simulink model "Modelo_sensores_reales_con_Kalman_discreto"  (R2021a)
settings: Solver=ode15s  StartTime=0.0  StopTime=7  FixedStep=0.0001  RelTol=1e-5
values from neighbouring files (symbols this model uses):
  A_d1 = (eye(4)+0.5*A*T_s)*(eye(4)-0.5*A*T_s)^(-1)    [Parametros.m]
  alpha = 0.5    [Parametros.m]
  Bu_d1 = B_d1(:,1)    [Parametros.m]
  C_d1 = C1    [Parametros.m]
  Cc = 1000    [Parametros.m]
  Cmax = 900    [Parametros.m]
  Cmin = 100    [Parametros.m]
  Du_d1 = D_d1(:,1)    [Parametros.m]
  Kc = 16000    [Parametros.m]
  Kr = 160000    [Parametros.m]
  Mc = 250    [Parametros.m]
  Mr = 45    [Parametros.m]
  R_d1 = R/T_s    [Parametros.m]
  T_s = 0.0001    [Parametros.m]
undefined symbols (not defined in the file or in its folder): Discrete, sigbuilder_block, Time
libraries: ctrlSharedLib x1
settings Model: Creator=fhlla  LastModifiedBy=fhlla
settings SolverCC: ZeroCrossAlgorithm=Adaptive
settings DebuggingCC: IgnoredZcDiagnostic=none

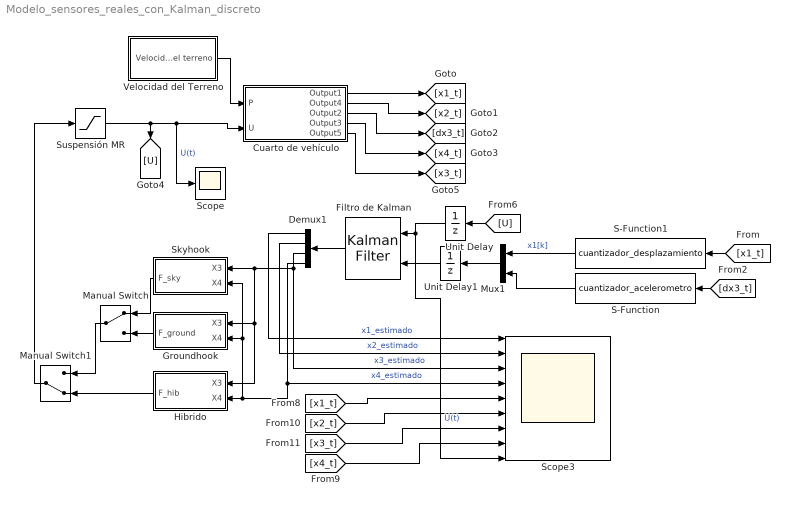
== system Modelo_sensores_reales_con_Kalman_discreto ==
  Cuarto de vehículo : Subsystem
  Demux1 : Demux
  Filtro de Kalman : ctrlSharedLib/Kalman Filter  TimeDomain=Discrete-Time  UseCurrentEstimator=on  ModelSource=Individual A, B, C, D matrices  ModelSourceVariable=ss(0.95,1,1,0,1)  A=A_d1  B=Bu_d1  C=C_d1  D=Du_d1  NumberOfStates=1  NumberOfInputs=1  NumberOfOutputs=1  InitialEstimateSource=Dialog  X0=0  P0=10  UseK=off  UseGH=off  NumberOfProcessNoiseInputs=1  G=1  TimeInvariantG=on  H=0  TimeInvariantH=on  Q=Q_d1  TimeInvariantQ=on  R=R_d1  TimeInvariantR=on  N=0  TimeInvariantN=on  AddInputPort=on  AddEnablePort=off  OutputEstimatedY=off  OutputP=off  Ts=T_s
  Groundhook : Subsystem
  Hibrido : Subsystem
  Manual Switch : ManualSwitch
  Manual Switch1 : ManualSwitch  CurrentSetting=0
  Mux1 : Mux  Inputs=2
  S-Function : S-Function  FunctionName=cuantizador_acelerometro  SFunctionDeploymentMode=off  EnableBusSupport=off
  S-Function1 : S-Function  FunctionName=cuantizador_desplazamiento  SFunctionDeploymentMode=off  EnableBusSupport=off
  Scope : Scope
  Scope3 : Scope  NumInputPorts=9
  Skyhook : Subsystem
  Suspensión MR : Saturate  UpperLimit=1500  LowerLimit=-1800
  Unit Delay : UnitDelay  SampleTime=T_s  HasFrameUpgradeWarning=on
  Unit Delay1 : UnitDelay  SampleTime=T_s  HasFrameUpgradeWarning=on
  Velocidad del Terreno : Subsystem  Tag=STV Subsys  LoadFcn=sigbuilder_block('load');  StartFcn=sigbuilder_block('start');  StopFcn=sigbuilder_block('stop');  ClipboardFcn=sigbuilder_block('clipboard');  mask(Sigbuilder block){tuvar=[0:10]}
      mask help: Simulink:masks:SigbuilderBlock_MD
      mask init:
      | if ~strcmp(get_param(bdroot(gcbh),'SimulationStatus'),'stopped') tuvar = sigbuilder_block('maskInit'); end
      settings: CopyFcn=sigbuilder_block('copy');  DeleteFcn=sigbuilder_block('delete');  ModelCloseFcn=sigbuilder_block('modelClose');  PreSaveFcn=sigbuilder_block('preSave');  PauseFcn=sigbuilder_block('pause');  ContinueFcn=sigbuilder_block('continue');  NameChangeFcn=sigbuilder_block('namechange');  OpenFcn=sigbuilder_block('open',[0 30 1024.5 488.25 ]);  CloseFcn=sigbuilder_block('close');
      mask Display: plot(0, 0, 100, 100,[2, 2, 32, 32, 2], [68, 8, 8, 68, 68],[32, 2], [38, 38], [32, 19, 2],[53, 60, 44], [32, 17, 17, 2],[16, 16, 31, 31]);txt = getActiveGroup(gcbh);text(2, 100, txt,'verticalAlignment', 'top');
  wires:
  Skyhook/1(F_sky) -> Manual Switch/1
  Groundhook/1(F_ground) -> Manual Switch/2
  Manual Switch/1 -> Manual Switch1/1
  Cuarto de vehículo/1(Output1) -> [x1_t]
  Cuarto de vehículo/2(Output4) -> [x2_t]
  Cuarto de vehículo/3(Output2) -> [dx3_t]
  S-Function1/1 -> Mux1/1  "x1[k]"
  [x1_t] -> S-Function1/1
  Cuarto de vehículo/5(Output5) -> [x3_t]
  Cuarto de vehículo/4(Output3) -> [x4_t]
  Velocidad del Terreno/1(Velocidad del terreno) -> Cuarto de vehículo/1(P)
  Hibrido/1(F_hib) -> Manual Switch1/2
  Manual Switch1/1 -> Suspensión MR/1
  [dx3_t] -> S-Function/1
  S-Function/1 -> Mux1/2
  Demux1/1 -> Scope3/1  "x1_estimado"
  Demux1/2 -> Scope3/2  "x2_estimado"
  Demux1/3 -> Scope3/3, Skyhook/1(X3), Hibrido/1(X3), Groundhook/1(X3)  "x3_estimado"
  Demux1/4 -> Hibrido/2(X4), Skyhook/2(X4), Groundhook/2(X4), Scope3/4  "x4_estimado"
  Mux1/1 -> Unit Delay1/1
  [x1_t] -> Scope3/5
  [x2_t] -> Scope3/6
  [x3_t] -> Scope3/7
  [x4_t] -> Scope3/8
  Filtro de Kalman/1 -> Demux1/1
  Unit Delay/1 -> Filtro de Kalman/1, Scope3/9  "U(t)"
  Unit Delay1/1 -> Filtro de Kalman/2
  [U] -> Unit Delay/1
  Suspensión MR/1 -> Cuarto de vehículo/2(U), Scope/1, [U]  "U(t)"

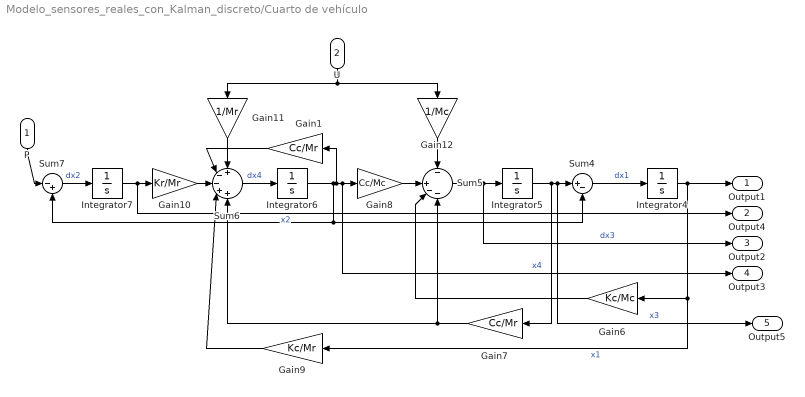
== system Modelo_sensores_reales_con_Kalman_discreto/Cuarto de vehículo ==
  P : Inport
  U : Inport  Port=2
  Gain1 : Gain  Gain=Cc/Mr
  Gain10 : Gain  Gain=Kr/Mr
  Gain11 : Gain  Gain=1/Mr
  Gain12 : Gain  Gain=1/Mc
  Gain6 : Gain  Gain=Kc/Mc
  Gain7 : Gain  Gain=Cc/Mr
  Gain8 : Gain  Gain=Cc/Mc
  Gain9 : Gain  Gain=Kc/Mr
  Integrator{4..7} (4 alike) : Integrator
  Sum4 : Sum  Inputs=|+-
  Sum5 : Sum  Inputs=-|+--
  Sum6 : Sum  Inputs=+--++
  Sum7 : Sum  Inputs=|-+
  Output1 : Outport
  Output4 : Outport  Port=2
  Output2 : Outport  Port=3
  Output3 : Outport  Port=4
  Output5 : Outport  Port=5
  wires:
  Sum7/1 -> Integrator7/1  "dx2"
  Sum6/1 -> Integrator6/1  "dx4"
  Gain9/1 -> Sum6/4
  Sum4/1 -> Integrator4/1  "dx1"
  U/1 -> Gain12/1, Gain11/1
  Sum5/1 -> Output2/1, Integrator5/1  "dx3"
  Integrator4/1 -> Gain9/1, Gain6/1, Output1/1  "x1"
  Gain10/1 -> Sum6/3
  Gain7/1 -> Sum6/5, Sum5/4
  P/1 -> Sum7/1
  Gain12/1 -> Sum5/1
  Integrator6/1 -> Gain1/1, Output3/1, Gain8/1, Sum7/2, Sum4/2  "x4"
  Integrator7/1 -> Output4/1, Gain10/1  "x2"
  Gain8/1 -> Sum5/2
  Integrator5/1 -> Output5/1, Sum4/1, Gain7/1  "x3"
  Gain1/1 -> Sum6/2
  Gain6/1 -> Sum5/3
  Gain11/1 -> Sum6/1

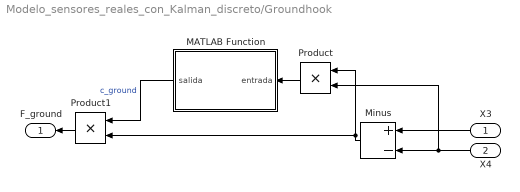
== system Modelo_sensores_reales_con_Kalman_discreto/Groundhook ==
  X3 : Inport
  X4 : Inport  Port=2
  MATLAB Function : MATLAB Function  TreatAsAtomicUnit=on
  Minus : Sum  Inputs=+-
  Product : Product
  Product1 : Product
  F_ground : Outport
  wires:
  Product/1 -> MATLAB Function/1(entrada)
  X4/1 -> Minus/2, Product/2
  Product1/1 -> F_ground/1
  Minus/1 -> Product1/2, Product/1
  MATLAB Function/1(salida) -> Product1/1  "c_ground"
  X3/1 -> Minus/1

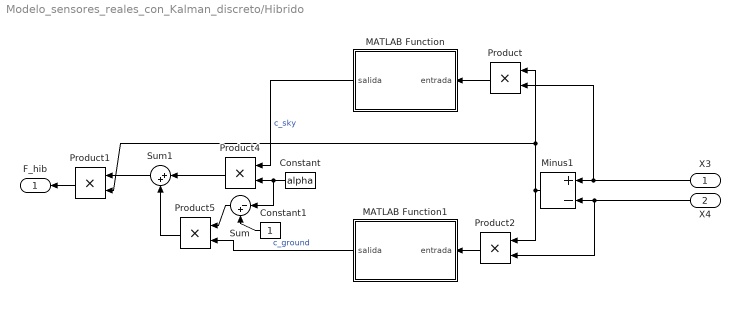
== system Modelo_sensores_reales_con_Kalman_discreto/Hibrido ==
  X3 : Inport
  X4 : Inport  Port=2
  Constant : Constant  Value=alpha
  Constant1 : Constant
  MATLAB Function : MATLAB Function  TreatAsAtomicUnit=on
  MATLAB Function1 : MATLAB Function  TreatAsAtomicUnit=on
  Minus1 : Sum  Inputs=+-
  Product{,1..2,4..5} (5 alike) : Product
  Sum : Sum  Inputs=|-+
  Sum1 : Sum  Inputs=|++
  F_hib : Outport
  wires:
  Product/1 -> MATLAB Function/1(entrada)
  MATLAB Function/1(salida) -> Product4/1  "c_sky"
  X3/1 -> Product/2, Minus1/1
  X4/1 -> Product2/2, Minus1/2
  Minus1/1 -> Product2/1, Product1/2, Product/1
  Product2/1 -> MATLAB Function1/1(entrada)
  MATLAB Function1/1(salida) -> Product5/2  "c_ground"
  Constant/1 -> Sum/1, Product4/2
  Constant1/1 -> Sum/2
  Sum/1 -> Product5/1
  Product5/1 -> Sum1/2
  Product4/1 -> Sum1/1
  Sum1/1 -> Product1/1
  Product1/1 -> F_hib/1

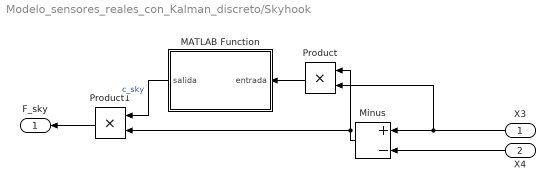
== system Modelo_sensores_reales_con_Kalman_discreto/Skyhook ==
  X3 : Inport
  X4 : Inport  Port=2
  MATLAB Function : MATLAB Function  TreatAsAtomicUnit=on
  Minus : Sum  Inputs=+-
  Product : Product
  Product1 : Product
  F_sky : Outport
  wires:
  Minus/1 -> Product1/2, Product/1
  Product/1 -> MATLAB Function/1(entrada)
  MATLAB Function/1(salida) -> Product1/1  "c_sky"
  Product1/1 -> F_sky/1
  X4/1 -> Minus/2
  X3/1 -> Product/2, Minus/1

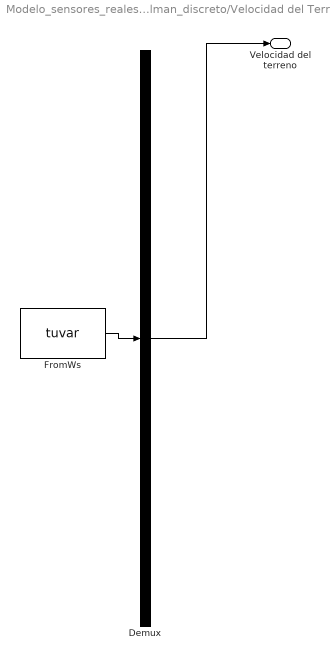
== system Modelo_sensores_reales_con_Kalman_discreto/Velocidad del Terreno ==
  Demux : Demux  Tag=STV Demux  Outputs=1
      settings: DisplayOption=none
  FromWs : FromWorkspace  Tag=STV FromWs  VariableName=tuvar
      SigBuilderData=|
      | common.afterFinalStr = 'Extrapolate'
      | common.sampleTime = 0
      | dataSet.timeRange = [0 11.5]
      | dataSet.name = 'Group 1'
      | sbobj.Groups.Name = 'Group 1'
      | sbobj.Groups.Signals.Name = 'Velocidad del terreno'
      | sbobj.Groups.Signals.XData = [0 1 1 1.0034 1.0034 1.0068 1.0068 1.0102 1.0102 11.5]
      | sbobj.Groups.Signals.YData = [0 0 14.71 14.71 0 0 -14.71 -14.71 0 0]
      | sbobj.Groups.TimeRange = [0 11.5]
  Velocidad del terreno : Outport  Tag=STV Outport
  wires:
  FromWs/1 -> Demux/1
  Demux/1 -> Velocidad del terreno/1

== matlab function Modelo_sensores_reales_con_Kalman_discreto/Groundhook/MATLAB Function ==
  data: entrada input; salida output; Cmax parameter; Cmin parameter
function salida = groundhook(entrada, Cmax, Cmin)
    if entrada<=0
        salida = Cmax % c_ground_max;
    else
        salida = Cmin % c_ground_min;
    end
end

== matlab function Modelo_sensores_reales_con_Kalman_discreto/Skyhook/MATLAB Function ==
  data: entrada input; salida output; Cmax parameter; Cmin parameter
function salida = skyhook(entrada, Cmax, Cmin)
    if entrada>=0
        salida = Cmax % c_sky_max;
    else
        salida = Cmin % c_sky_min;   200
    end
end

== matlab function Modelo_sensores_reales_con_Kalman_discreto/Hibrido/MATLAB Function ==
  data: entrada input; salida output; Cmax parameter; Cmin parameter
function salida = skyhook(entrada, Cmax, Cmin)
    if entrada>=0
        salida = Cmax % c_sky_max;
    else
        salida = Cmin % c_sky_min;   200
    end
end

== matlab function Modelo_sensores_reales_con_Kalman_discreto/Hibrido/MATLAB Function1 ==
  data: entrada input; salida output; Cmax parameter; Cmin parameter
function salida = groundhook(entrada, Cmax, Cmin)
    if entrada<=0
        salida = Cmax % c_ground_max;
    else
        salida = Cmin % c_ground_min;
    end
end
